simulink model "mechanical_model_step_input"  (R2019b)
settings: Solver=FixedStepAuto  StartTime=0.0  StopTime=60  FixedStep=1e-3  RelTol=1e-3
undefined symbols (not defined in the file or in its folder): amplVstep, tf2_1, tf2_2
settings Model: Creator=Guido  LastModifiedBy=pietr

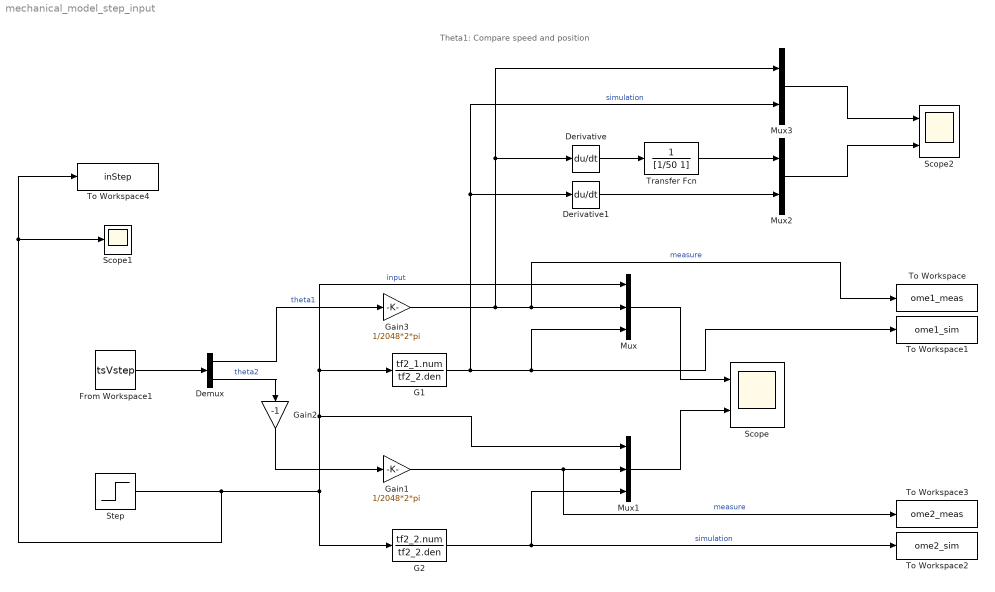
== system mechanical_model_step_input ==
  note: Theta1: Compare speed and position
  Demux : Demux  Outputs=2
  Derivative : Derivative  CoefficientInTFapproximation=100
  Derivative1 : Derivative  CoefficientInTFapproximation=100
  From Workspace1 : FromWorkspace  VariableName=tsVstep  SampleTime=0
  G1 : TransferFcn  Numerator=tf2_1.num  Denominator=tf2_2.den
  G2 : TransferFcn  Numerator=tf2_2.num  Denominator=tf2_2.den
  Gain1 : Gain  Gain=1/2048*2*pi
  Gain2 : Gain  Gain=-1
  Gain3 : Gain  Gain=1/2048*2*pi
  Mux : Mux  Inputs=3
  Mux1 : Mux  Inputs=3
  Mux2 : Mux  Inputs=2
  Mux3 : Mux  Inputs=2
  Scope : Scope  NumInputPorts=2
  Scope1 : Scope
  Scope2 : Scope  NumInputPorts=2
  Step : Step  After=amplVstep  SampleTime=0
  To Workspace : ToWorkspace  VariableName=ome1_meas  SampleTime=-1
      settings: Save2DSignal=2-D array (concatenate along first dimension)
  To Workspace1 : ToWorkspace  VariableName=ome1_sim  SampleTime=-1
      settings: Save2DSignal=2-D array (concatenate along first dimension)
  To Workspace2 : ToWorkspace  VariableName=ome2_sim  SampleTime=-1
      settings: Save2DSignal=2-D array (concatenate along first dimension)
  To Workspace3 : ToWorkspace  VariableName=ome2_meas  SampleTime=-1
      settings: Save2DSignal=2-D array (concatenate along first dimension)
  To Workspace4 : ToWorkspace  VariableName=inStep  SaveFormat=Timeseries  SampleTime=-1
  Transfer Fcn : TransferFcn  Denominator=[1/50 1]
  wires:
  Gain1/1 -> Mux1/2, To Workspace3/1  "measure"
  Demux/1 -> Gain3/1  "theta1"
  Demux/2 -> Gain2/1  "theta2"
  Mux/1 -> Scope/1
  Mux1/1 -> Scope/2
  Gain2/1 -> Gain1/1
  Gain3/1 -> Mux/2, To Workspace/1, Mux3/1, Derivative/1  "measure"
  G1/1 -> Mux/3, To Workspace1/1, Mux3/2, Derivative1/1  "simulation"
  G2/1 -> Mux1/3, To Workspace2/1  "simulation"
  From Workspace1/1 -> Demux/1
  Step/1 -> Scope1/1, To Workspace4/1, G2/1, Mux1/1, G1/1, Mux/1  "input"
  Derivative1/1 -> Mux2/2
  Derivative/1 -> Transfer Fcn/1
  Transfer Fcn/1 -> Mux2/1
  Mux3/1 -> Scope2/1
  Mux2/1 -> Scope2/2
